simulink model "gm_inc_enc_v25_vnl"  (R2022a)
settings: Solver=FixedStepDiscrete  StartTime=0.0  StopTime=SimulationsDauer  RelTol=1e-3
undefined symbols (not defined in the file or in its folder): DiscIntNeverNeededParam, f_ISR, IncPerTurn, inital_zero_speed_timeout, n_max, OmegaPerOverSampl, Periode, Phase_Delay_A, Phase_Delay_B, PolePair, QuadratureFactor, reciprocal_iterations, T_fpga, T_mech
libraries: simulink x19, hdlsllib x11, hdlmdlgenlib x4, dspsrcs4 x3, dspswit3 x2, spsEdgeDetectorLib x2, simulink_extras x1
(part 2 of 4)

== system gm_inc_enc_v25_vnl/Compare/Assert_theta_el ==
  cosim : Inport
  dut : Inport  Port=2
  AssertEq : Assertion  StopWhenAssertionFail=off
  Compare To Zero : simulink/Logic and Bit Operations/Compare To Zero  relop===  OutDataTypeStr=boolean
  Relational Operator : RelationalOperator  Operator===  OutDataTypeStr=boolean  InputSameDT=off
  compare: theta_el : Scope  NumInputPorts=3
  wires:
  Compare To Zero/1 -> compare: theta_el/3  "err"
  Relational Operator/1 -> Compare To Zero/1, AssertEq/1
  cosim/1 -> compare: theta_el/1, Relational Operator/1  "cosim"
  dut/1 -> compare: theta_el/2, Relational Operator/2  "dut ref"

== system gm_inc_enc_v25_vnl/Compare/Assert_theta_el_AXI4 ==
  cosim : Inport
  dut : Inport  Port=2
  AssertEq : Assertion  StopWhenAssertionFail=off
  Compare To Zero : simulink/Logic and Bit Operations/Compare To Zero  relop===  OutDataTypeStr=boolean
  Relational Operator : RelationalOperator  Operator===  OutDataTypeStr=boolean  InputSameDT=off
  compare: theta_el_AXI4 : Scope  NumInputPorts=3
  wires:
  Compare To Zero/1 -> compare: theta_el_AXI4/3  "err"
  Relational Operator/1 -> Compare To Zero/1, AssertEq/1
  cosim/1 -> compare: theta_el_AXI4/1, Relational Operator/1  "cosim"
  dut/1 -> compare: theta_el_AXI4/2, Relational Operator/2  "dut ref"

== system gm_inc_enc_v25_vnl/Compare/Assert_timeout_active ==
  cosim : Inport
  dut : Inport  Port=2
  AssertEq : Assertion  StopWhenAssertionFail=off
  Compare To Zero : simulink/Logic and Bit Operations/Compare To Zero  relop===  OutDataTypeStr=boolean
  Relational Operator : RelationalOperator  Operator===  OutDataTypeStr=boolean  InputSameDT=off
  compare: timeout_active : Scope  NumInputPorts=3
  wires:
  Compare To Zero/1 -> compare: timeout_active/3  "err"
  Relational Operator/1 -> Compare To Zero/1, AssertEq/1
  cosim/1 -> compare: timeout_active/1, Relational Operator/1  "cosim"
  dut/1 -> compare: timeout_active/2, Relational Operator/2  "dut ref"

== system gm_inc_enc_v25_vnl/Compare/CleanupScopes ==

== system gm_inc_enc_v25_vnl/Compare/Enable ==

== system gm_inc_enc_v25_vnl/IncEnc_V25/Counter ==
  note: 1 for one cycle if edge recognized
  note: Reset
  Enable_ctr : Inport  OutDataTypeStr=boolean  PortDimensions=1  SampleTime=1e-08
  I_line : Inport  Port=2  OutDataTypeStr=boolean  PortDimensions=1  SampleTime=1e-08
  Detec_edge : Sum  Inputs=+-  AccumDataTypeStr=int8  OutDataTypeStr=int8  SampleTime=1e-08
  Reset_flag : Sum  Inputs=+-  AccumDataTypeStr=uint8  OutDataTypeStr=uint8  SampleTime=1e-08
  reset_old : Delay  DelayLength=double(1)  InitialCondition=0  SampleTime=1e-08
  reset_old1 : Delay  DelayLength=double(1)  InitialCondition=0  SampleTime=1e-08
  reset_old_switch : Switch  Criteria=u2 ~= 0  Threshold=double(0)  OutDataTypeStr=boolean  SampleTime=1e-08  SaturateOnIntegerOverflow=off  InputSameDT=off
  reset_old_switch1 : Switch  Criteria=u2 ~= 0  Threshold=double(0)  OutDataTypeStr=boolean  SampleTime=1e-08  SaturateOnIntegerOverflow=off  InputSameDT=off
  Edge : Outport  SampleTime=1e-08  VectorParamsAs1DForOutWhenUnconnected=off
  Reset : Outport  Port=2  SampleTime=1e-08  VectorParamsAs1DForOutWhenUnconnected=off
  wires:
  reset_old/1 -> Reset_flag/2, reset_old_switch/3
  reset_old_switch/1 -> reset_old/1
  reset_old1/1 -> Detec_edge/2, reset_old_switch1/3
  reset_old_switch1/1 -> reset_old1/1
  Reset_flag/1 -> reset_old_switch/2, Reset/1
  Detec_edge/1 -> reset_old_switch1/2, Edge/1
  I_line/1 -> reset_old_switch/1, Reset_flag/1
  Enable_ctr/1 -> reset_old_switch1/1, Detec_edge/1

== system gm_inc_enc_v25_vnl/IncEnc_V25/Counter_position ==
  note: Count
  note: Check if count is to big 0-Increments
  note: Check if count is to small
  Edge : Inport  OutDataTypeStr=int8  PortDimensions=1  SampleTime=1e-08
  Reset : Inport  Port=2  OutDataTypeStr=uint8  PortDimensions=1  SampleTime=1e-08
  IncsPerTurn : Inport  Port=3  OutDataTypeStr=uint16  PortDimensions=1  SampleTime=1e-08
  Dir : Inport  Port=4  OutDataTypeStr=fixdt(1, 4, 0)  PortDimensions=1  SampleTime=1e-08
  Add1 : Sum  AccumDataTypeStr=int16  OutDataTypeStr=int16  SampleTime=1e-08
  Constant1 : Constant  Value=0  OutDataTypeStr=int16  SampleTime=1e-08
  Constant2 : Constant  OutDataTypeStr=int16  SampleTime=1e-08
  Constant3 : Constant  Value=0  OutDataTypeStr=int16  SampleTime=1e-08
  Constant5 : Constant  Value=-1  OutDataTypeStr=int16  SampleTime=1e-08
  Relational Operator : RelationalOperator  Operator=>  OutDataTypeStr=boolean  SampleTime=1e-08  InputSameDT=off
  Relational Operator1 : RelationalOperator  Operator=<=  OutDataTypeStr=boolean  SampleTime=1e-08  InputSameDT=off
  Resett_switch1 : Switch  Criteria=u2 ~= 0  Threshold=double(0)  OutDataTypeStr=uint16  SampleTime=1e-08  SaturateOnIntegerOverflow=off  InputSameDT=off
  Resett_switch2 : Switch  Criteria=u2 ~= 0  Threshold=double(0)  OutDataTypeStr=int16  SampleTime=1e-08  SaturateOnIntegerOverflow=off  InputSameDT=off
  Resett_switch3 : Switch  Criteria=u2 ~= 0  Threshold=double(0)  OutDataTypeStr=int16  SampleTime=1e-08  SaturateOnIntegerOverflow=off  InputSameDT=off
  only_use_for_neg_speed : Switch  Threshold=double(1)  OutDataTypeStr=int16  SampleTime=1e-08  SaturateOnIntegerOverflow=off  InputSameDT=off
  reset_old{1..6} (6 alike) : Delay  DelayLength=double(1)  InitialCondition=0  SampleTime=1e-08
  speed_old_switch1 : Switch  Criteria=u2 ~= 0  Threshold=double(0)  OutDataTypeStr=int16  SampleTime=1e-08  SaturateOnIntegerOverflow=off  InputSameDT=off
  speed_old_switch2 : Switch  Threshold=double(1)  OutDataTypeStr=int16  SampleTime=1e-08  SaturateOnIntegerOverflow=off  InputSameDT=off
  count : Outport  SampleTime=1e-08  VectorParamsAs1DForOutWhenUnconnected=off
  wires:
  reset_old3/1 -> Resett_switch1/2
  Relational Operator/1 -> reset_old3/1
  Resett_switch3/1 -> Relational Operator1/1, Resett_switch1/3
  only_use_for_neg_speed/1 -> Resett_switch3/2
  reset_old2/1 -> only_use_for_neg_speed/3
  Relational Operator1/1 -> reset_old2/1
  reset_old1/1 -> Add1/2
  Add1/1 -> Resett_switch2/3
  Resett_switch2/1 -> Resett_switch3/3
  speed_old_switch2/1 -> reset_old4/1
  speed_old_switch1/1 -> Add1/1
  reset_old6/1 -> only_use_for_neg_speed/2, speed_old_switch2/2
  reset_old5/1 -> Resett_switch3/1, Relational Operator/2
  reset_old4/1 -> speed_old_switch1/1
  Resett_switch1/1 -> Relational Operator/1, reset_old1/1, count/1
  Constant5/1 -> speed_old_switch2/3
  Constant3/1 -> speed_old_switch1/3
  Constant2/1 -> speed_old_switch2/1
  Constant1/1 -> only_use_for_neg_speed/1, Resett_switch2/1, Resett_switch1/1, Relational Operator1/2
  Dir/1 -> reset_old6/1
  IncsPerTurn/1 -> reset_old5/1
  Reset/1 -> Resett_switch2/2
  Edge/1 -> speed_old_switch1/2

== system gm_inc_enc_v25_vnl/IncEnc_V25/Counter_theta_ele ==
  note: Count
  note: Check if count is to small
  Edge : Inport  OutDataTypeStr=int8  PortDimensions=1  SampleTime=1e-08
  Reset : Inport  Port=2  OutDataTypeStr=uint8  PortDimensions=1  SampleTime=1e-08
  IncsPerTurn : Inport  Port=3  OutDataTypeStr=uint16  PortDimensions=1  SampleTime=1e-08
  Dir : Inport  Port=4  OutDataTypeStr=fixdt(1, 4, 0)  PortDimensions=1  SampleTime=1e-08
  Add1 : Sum  AccumDataTypeStr=int16  OutDataTypeStr=int16  SampleTime=1e-08
  Constant1 : Constant  Value=0  OutDataTypeStr=int16  SampleTime=1e-08
  Constant2 : Constant  OutDataTypeStr=int16  SampleTime=1e-08
  Constant3 : Constant  Value=0  OutDataTypeStr=int16  SampleTime=1e-08
  Constant5 : Constant  Value=-1  OutDataTypeStr=int16  SampleTime=1e-08
  Relational Operator : RelationalOperator  Operator=>  OutDataTypeStr=boolean  SampleTime=1e-08  InputSameDT=off
  Relational Operator1 : RelationalOperator  Operator=<=  OutDataTypeStr=boolean  SampleTime=1e-08  InputSameDT=off
  Reset_switch3 : Switch  Criteria=u2 ~= 0  Threshold=double(0)  OutDataTypeStr=int16  SampleTime=1e-08  SaturateOnIntegerOverflow=off  InputSameDT=off
  Resett_switch1 : Switch  Criteria=u2 ~= 0  Threshold=double(0)  OutDataTypeStr=int16  SampleTime=1e-08  SaturateOnIntegerOverflow=off  InputSameDT=off
  Resett_switch2 : Switch  Criteria=u2 ~= 0  Threshold=double(0)  OutDataTypeStr=int16  SampleTime=1e-08  SaturateOnIntegerOverflow=off  InputSameDT=off
  only_use_for_neg_speed : Switch  Threshold=double(1)  OutDataTypeStr=int16  SampleTime=1e-08  SaturateOnIntegerOverflow=off  InputSameDT=off
  reset_old{1..6} (6 alike) : Delay  DelayLength=double(1)  InitialCondition=0  SampleTime=1e-08
  speed_old_switch1 : Switch  Criteria=u2 ~= 0  Threshold=double(0)  OutDataTypeStr=int16  SampleTime=1e-08  SaturateOnIntegerOverflow=off  InputSameDT=off
  speed_old_switch2 : Switch  Threshold=double(1)  OutDataTypeStr=int16  SampleTime=1e-08  SaturateOnIntegerOverflow=off  InputSameDT=off
  count : Outport  SampleTime=1e-08  VectorParamsAs1DForOutWhenUnconnected=off
  wires:
  reset_old3/1 -> Resett_switch1/2
  Relational Operator/1 -> reset_old3/1
  Reset_switch3/1 -> Relational Operator1/1, Resett_switch1/3
  only_use_for_neg_speed/1 -> Reset_switch3/2
  reset_old2/1 -> only_use_for_neg_speed/3
  Relational Operator1/1 -> reset_old2/1
  reset_old6/1 -> Add1/2
  Add1/1 -> Resett_switch2/3
  Resett_switch2/1 -> Reset_switch3/3
  speed_old_switch2/1 -> reset_old4/1
  speed_old_switch1/1 -> Add1/1
  reset_old5/1 -> only_use_for_neg_speed/2, speed_old_switch2/2
  reset_old4/1 -> speed_old_switch1/1
  reset_old1/1 -> Reset_switch3/1, Relational Operator/2
  Resett_switch1/1 -> Relational Operator/1, reset_old6/1, count/1
  Constant5/1 -> speed_old_switch2/3
  Constant3/1 -> speed_old_switch1/3
  Constant2/1 -> speed_old_switch2/1
  Constant1/1 -> only_use_for_neg_speed/1, Resett_switch2/1, Resett_switch1/1, Relational Operator1/2
  Dir/1 -> reset_old5/1
  IncsPerTurn/1 -> reset_old1/1
  Reset/1 -> Resett_switch2/2
  Edge/1 -> speed_old_switch1/2

== system gm_inc_enc_v25_vnl/IncEnc_V25/Direction ==
  A : Inport  OutDataTypeStr=boolean  PortDimensions=1  SampleTime=1e-08
  B : Inport  Port=2  OutDataTypeStr=boolean  PortDimensions=1  SampleTime=1e-08
  Add : Sum  Inputs=+-  AccumDataTypeStr=fixdt(1, 4, 0)  OutDataTypeStr=fixdt(1, 4, 0)  SampleTime=1e-08
  Add1 : Sum  Inputs=+-  AccumDataTypeStr=fixdt(1, 4, 0)  OutDataTypeStr=fixdt(1, 4, 0)  SampleTime=1e-08
  Add2 : Sum  AccumDataTypeStr=fixdt(1, 4, 0)  OutDataTypeStr=fixdt(1, 4, 0)  SampleTime=1e-08
  Change : Sum  AccumDataTypeStr=fixdt(1, 4, 0)  OutDataTypeStr=fixdt(1, 4, 0)  SampleTime=1e-08
  Change1 : Delay  DelayLength=double(1)  InitialCondition=0  SampleTime=1e-08
  Save_Direction : Switch  Criteria=u2 ~= 0  Threshold=double(0)  OutDataTypeStr=fixdt(1, 4, 0)  SampleTime=1e-08  SaturateOnIntegerOverflow=off  InputSameDT=off
  T_count_switch : Switch  Threshold=double(1)  OutDataTypeStr=fixdt(1, 4, 0)  SampleTime=1e-08  SaturateOnIntegerOverflow=off  InputSameDT=off
  TrnLeft : Sum  Inputs=+-  AccumDataTypeStr=fixdt(1, 4, 0)  OutDataTypeStr=fixdt(1, 4, 0)  SampleTime=1e-08
  TrnRight : Sum  Inputs=+-  AccumDataTypeStr=fixdt(1, 4, 0)  OutDataTypeStr=fixdt(1, 4, 0)  SampleTime=1e-08
  TurnLeft : Constant  Value=-1  OutDataTypeStr=fixdt(1, 4, 0)  SampleTime=1e-08
  TurnRight : Constant  OutDataTypeStr=fixdt(1, 4, 0)  SampleTime=1e-08
  count_old : Delay  DelayLength=double(1)  InitialCondition=0  SampleTime=1e-08
  count_old1 : Delay  DelayLength=double(1)  InitialCondition=0  SampleTime=1e-08
  count_old2 : Delay  DelayLength=double(1)  InitialCondition=0  SampleTime=1e-08
  count_old_switch : Switch  Criteria=u2 ~= 0  Threshold=double(0)  OutDataTypeStr=boolean  SampleTime=1e-08  SaturateOnIntegerOverflow=off  InputSameDT=off
  count_old_switch1 : Switch  Criteria=u2 ~= 0  Threshold=double(0)  OutDataTypeStr=boolean  SampleTime=1e-08  SaturateOnIntegerOverflow=off  InputSameDT=off
  new_value : Delay  DelayLength=double(1)  InitialCondition=0  SampleTime=1e-08
  nothing : Constant  Value=0  OutDataTypeStr=fixdt(1, 4, 0)  SampleTime=1e-08
  nothing1 : Constant  Value=0  OutDataTypeStr=fixdt(1, 4, 0)  SampleTime=1e-08
  speed_old_switch : Switch  Threshold=double(1)  OutDataTypeStr=fixdt(1, 4, 0)  SampleTime=1e-08  SaturateOnIntegerOverflow=off  InputSameDT=off
  Dir : Outport  SampleTime=1e-08  VectorParamsAs1DForOutWhenUnconnected=off
  wires:
  Save_Direction/1 -> count_old2/1
  count_old1/1 -> Add1/2, count_old_switch1/3
  count_old_switch1/1 -> count_old1/1
  count_old/1 -> Add/2, count_old_switch/3
  count_old_switch/1 -> count_old/1
  speed_old_switch/1 -> Add2/2, Change/2
  nothing1/1 -> T_count_switch/3
  nothing/1 -> speed_old_switch/3
  new_value/1 -> Save_Direction/1
  count_old2/1 -> Save_Direction/3, Dir/1
  TurnRight/1 -> T_count_switch/1
  TurnLeft/1 -> speed_old_switch/1
  TrnRight/1 -> T_count_switch/2
  TrnLeft/1 -> speed_old_switch/2
  T_count_switch/1 -> Add2/1, Change/1
  Change1/1 -> Save_Direction/2
  Change/1 -> Change1/1
  Add2/1 -> new_value/1
  Add1/1 -> count_old_switch1/2, TrnLeft/1
  Add/1 -> count_old_switch/2, TrnRight/1
  B/1 -> count_old_switch1/1, Add1/1, TrnRight/2
  A/1 -> count_old_switch/1, Add/1, TrnLeft/2

== system gm_inc_enc_v25_vnl/IncEnc_V25/count_lines ==
  note: Set new counter value
  note: Check if count is to big in order to safe for value overflow
  note: Count
  Edge : Inport  OutDataTypeStr=int8  PortDimensions=1  SampleTime=1e-08
  Reset : Inport  Port=2  OutDataTypeStr=boolean  PortDimensions=1  SampleTime=1e-08
  IncsPerTurn : Inport  Port=3  OutDataTypeStr=uint16  PortDimensions=1  SampleTime=1e-08
  Add1 : Sum  AccumDataTypeStr=int16  OutDataTypeStr=int16  SampleTime=1e-08
  Constant1 : Constant  Value=0  OutDataTypeStr=int16  SampleTime=1e-08
  Constant2 : Constant  OutDataTypeStr=int16  SampleTime=1e-08
  Constant3 : Constant  Value=0  OutDataTypeStr=int16  SampleTime=1e-08
  Constant4 : Constant  Value=10  OutDataTypeStr=int16  SampleTime=1e-08
  Relational Operator : RelationalOperator  Operator=>  OutDataTypeStr=boolean  SampleTime=1e-08  InputSameDT=off
  Reset_when_overflow : Sum  AccumDataTypeStr=fixdt(1, 18, 0)  OutDataTypeStr=int16  SampleTime=1e-08
  Resett_switch1 : Switch  Criteria=u2 ~= 0  Threshold=double(0)  OutDataTypeStr=int16  SampleTime=1e-08  SaturateOnIntegerOverflow=off  InputSameDT=off
  Resett_switch2 : Switch  Criteria=u2 ~= 0  Threshold=double(0)  OutDataTypeStr=int16  SampleTime=1e-08  SaturateOnIntegerOverflow=off  InputSameDT=off
  reset_old{1,3..5} (4 alike) : Delay  DelayLength=double(1)  InitialCondition=0  SampleTime=1e-08
  reset_old_switch1 : Switch  Criteria=u2 ~= 0  Threshold=double(0)  OutDataTypeStr=int16  SampleTime=1e-08  SaturateOnIntegerOverflow=off  InputSameDT=off
  speed_old_switch1 : Switch  Criteria=u2 ~= 0  Threshold=double(0)  OutDataTypeStr=int16  SampleTime=1e-08  SaturateOnIntegerOverflow=off  InputSameDT=off
  count : Outport  SampleTime=1e-08  VectorParamsAs1DForOutWhenUnconnected=off
  wires:
  reset_old1/1 -> reset_old_switch1/3
  Resett_switch1/1 -> reset_old3/1
  Relational Operator/1 -> Resett_switch1/2
  Add1/1 -> Resett_switch2/3
  Resett_switch2/1 -> Resett_switch1/3
  speed_old_switch1/1 -> Add1/1
  reset_old_switch1/1 -> reset_old1/1, count/1
  reset_old5/1 -> Relational Operator/2
  reset_old4/1 -> speed_old_switch1/1
  reset_old3/1 -> reset_old_switch1/1, Relational Operator/1, Add1/2
  Reset_when_overflow/1 -> reset_old5/1
  Constant4/1 -> Reset_when_overflow/1
  Constant3/1 -> speed_old_switch1/3
  Constant2/1 -> reset_old4/1
  Constant1/1 -> Resett_switch2/1, Resett_switch1/1
  IncsPerTurn/1 -> Reset_when_overflow/2
  Reset/1 -> reset_old_switch1/2, Resett_switch2/2
  Edge/1 -> speed_old_switch1/2

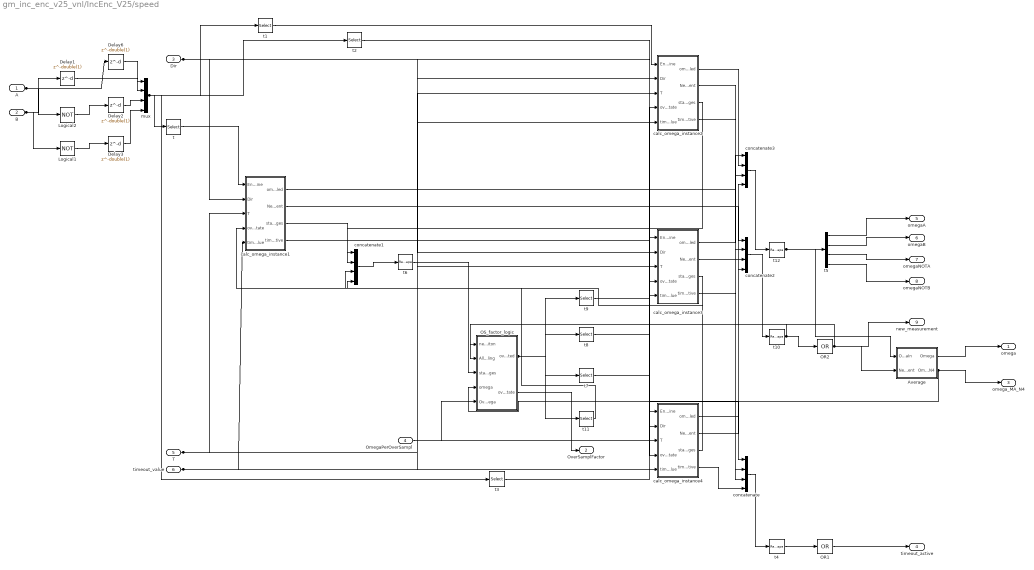
== system gm_inc_enc_v25_vnl/IncEnc_V25/speed ==
  A : Inport  OutDataTypeStr=boolean  PortDimensions=1  SampleTime=1e-08
  B : Inport  Port=2  OutDataTypeStr=boolean  PortDimensions=1  SampleTime=1e-08
  Dir : Inport  Port=3  OutDataTypeStr=fixdt(1, 4, 0)  PortDimensions=1  SampleTime=1e-08
  OmegaPerOverSampl : Inport  Port=4  OutDataTypeStr=fixdt(1, 24, 11)  PortDimensions=1  SampleTime=1e-08
  T : Inport  Port=5  OutDataTypeStr=fixdt(1, 38, 32)  PortDimensions=1  SampleTime=1e-08
  timeout_value : Inport  Port=6  OutDataTypeStr=uint32  PortDimensions=1  SampleTime=1e-08
  Average : Subsystem
  Delay{1..3,6} (4 alike) : Delay  DelayLength=double(1)  InitialCondition=0  SampleTime=1e-08
  Logical1 : Logic  Operator=NOT  Inputs=1  AllPortsSameDT=off  OutDataTypeStr=boolean  SampleTime=1e-08
  Logical2 : Logic  Operator=NOT  Inputs=1  AllPortsSameDT=off  OutDataTypeStr=boolean  SampleTime=1e-08
  OR1 : Logic  Operator=OR  Inputs=1  AllPortsSameDT=off  OutDataTypeStr=boolean  SampleTime=1e-08
  OR2 : Logic  Operator=OR  Inputs=1  AllPortsSameDT=off  OutDataTypeStr=boolean  SampleTime=1e-08
  OS_factor_logic : Subsystem
  calc_omega_instance1 : Subsystem
  calc_omega_instance2 : Subsystem
  calc_omega_instance3 : Subsystem
  calc_omega_instance4 : Subsystem
  concatenate{,1..3} (4 alike) : Concatenate  NumInputs=4
  mux : Mux
  t : Selector  SampleTime=1e-08  IndexOptions=Index vector (dialog)  Indices=double(1)  OutputSizes=1
  t1 : Selector  SampleTime=1e-08  IndexOptions=Index vector (dialog)  Indices=double(2)  OutputSizes=1
  t{4,6,10,12} (4 alike) : Reshape
  t11 : Selector  SampleTime=1e-08  IndexOptions=Index vector (dialog)  Indices=double(1)  OutputSizes=1
  t2 : Selector  SampleTime=1e-08  IndexOptions=Index vector (dialog)  Indices=double(3)  OutputSizes=1
  t3 : Selector  SampleTime=1e-08  IndexOptions=Index vector (dialog)  Indices=double(4)  OutputSizes=1
  t5 : Demux
  t7 : Selector  SampleTime=1e-08  IndexOptions=Index vector (dialog)  Indices=double(4)  OutputSizes=1
  t8 : Selector  SampleTime=1e-08  IndexOptions=Index vector (dialog)  Indices=double(3)  OutputSizes=1
  t9 : Selector  SampleTime=1e-08  IndexOptions=Index vector (dialog)  Indices=double(2)  OutputSizes=1
  omega : Outport  SampleTime=1e-08  VectorParamsAs1DForOutWhenUnconnected=off
  OverSamplFactor : Outport  Port=2  SampleTime=1e-08
  omega_MA_N4 : Outport  Port=3  SampleTime=1e-08  VectorParamsAs1DForOutWhenUnconnected=off
  timeout_active : Outport  Port=4  OutDataTypeStr=boolean  SampleTime=1e-08  VectorParamsAs1DForOutWhenUnconnected=off
  omegaA : Outport  Port=5  SampleTime=1e-08  VectorParamsAs1DForOutWhenUnconnected=off
  omegaB : Outport  Port=6  SampleTime=1e-08  VectorParamsAs1DForOutWhenUnconnected=off
  omegaNOTA : Outport  Port=7  SampleTime=1e-08  VectorParamsAs1DForOutWhenUnconnected=off
  omegaNOTB : Outport  Port=8  SampleTime=1e-08  VectorParamsAs1DForOutWhenUnconnected=off
  new_measurement : Outport  Port=9  OutDataTypeStr=boolean  SampleTime=1e-08  VectorParamsAs1DForOutWhenUnconnected=off
  wires:
  concatenate3/1 -> t12/1
  calc_omega_instance1/3(state_count_edges) -> concatenate1/1
  calc_omega_instance1/2(NewMeasurement) -> concatenate2/1
  calc_omega_instance1/1(omega_oversampled) -> concatenate3/1
  t11/1 -> calc_omega_instance1/4(oversampling_state)
  OS_factor_logic/1(oversampling_adjusted) -> t11/1, t9/1, t8/1, t7/1
  t10/1 -> OS_factor_logic/1(new_transisiton), OR2/1
  concatenate2/1 -> t10/1
  calc_omega_instance2/3(state_count_edges) -> concatenate1/2
  calc_omega_instance2/2(NewMeasurement) -> concatenate2/2
  calc_omega_instance2/1(omega_oversampled) -> concatenate3/2
  t9/1 -> calc_omega_instance2/4(oversampling_state)
  calc_omega_instance3/3(state_count_edges) -> concatenate1/3
  calc_omega_instance3/2(NewMeasurement) -> concatenate2/3
  calc_omega_instance3/1(omega_oversampled) -> concatenate3/3
  t8/1 -> calc_omega_instance3/4(oversampling_state)
  calc_omega_instance4/3(state_count_edges) -> concatenate1/4
  calc_omega_instance4/2(NewMeasurement) -> concatenate2/4
  calc_omega_instance4/1(omega_oversampled) -> concatenate3/4
  t7/1 -> calc_omega_instance4/4(oversampling_state)
  t6/1 -> OS_factor_logic/3(state_edges)
  concatenate1/1 -> t6/1
  t5/4 -> omegaNOTB/1
  t5/3 -> omegaNOTA/1
  t5/2 -> omegaB/1
  t5/1 -> omegaA/1
  calc_omega_instance4/4(timeout_active) -> concatenate/4
  calc_omega_instance3/4(timeout_active) -> concatenate/3
  calc_omega_instance2/4(timeout_active) -> concatenate/2
  calc_omega_instance1/4(timeout_active) -> concatenate/1
  concatenate/1 -> t4/1
  t3/1 -> calc_omega_instance4/1(Encoder Line)
  t2/1 -> calc_omega_instance3/1(Encoder Line)
  t1/1 -> calc_omega_instance2/1(Encoder Line)
  t/1 -> calc_omega_instance1/1(Encoder Line)
  t4/1 -> OR1/1
  t12/1 -> Average/1("OmegaIn "), t5/1
  OS_factor_logic/2(oversampling_state) -> OverSamplFactor/1
  OR2/1 -> OS_factor_logic/2(Allow_ToCheckOversampling), Average/2(NewMeasurement), new_measurement/1
  OR1/1 -> timeout_active/1
  mux/1 -> t/1, t1/1, t2/1, t3/1
  Logical2/1 -> Delay2/1
  Logical1/1 -> Delay3/1
  Delay6/1 -> mux/1
  Delay3/1 -> mux/4
  Delay2/1 -> mux/3
  Delay1/1 -> mux/2
  Average/2(OmegaOut_MA_N4) -> OS_factor_logic/4(omega), omega_MA_N4/1
  Average/1(Omega) -> omega/1
  timeout_value/1 -> calc_omega_instance4/5(timeout_value), calc_omega_instance3/5(timeout_value), calc_omega_instance2/5(timeout_value), calc_omega_instance1/5(timeout_value)
  T/1 -> calc_omega_instance4/3(T), calc_omega_instance3/3(T), calc_omega_instance2/3(T), calc_omega_instance1/3(T)
  OmegaPerOverSampl/1 -> OS_factor_logic/5(OverSamplOmega)
  Dir/1 -> calc_omega_instance4/2(Dir), calc_omega_instance3/2(Dir), calc_omega_instance2/2(Dir), calc_omega_instance1/2(Dir)
  B/1 -> Delay1/1, Logical1/1
  A/1 -> Delay6/1, Logical2/1

== system gm_inc_enc_v25_vnl/IncEnc_V25_vnl/Counter ==
  note: Reset
  note: 1 for one cycle if edge recognized
  Enable_ctr : Inport
  I_line : Inport  Port=2
  Detec_edge : Sum  Inputs=+-  AccumDataTypeStr=int8  OutDataTypeStr=int8
  Reset_flag : Sum  Inputs=+-  AccumDataTypeStr=uint8  OutDataTypeStr=uint8
  reset_old : Delay  DelayLength=1
  reset_old1 : Delay  DelayLength=1
  reset_old_switch : Switch  Criteria=u2 ~= 0  SaturateOnIntegerOverflow=off  InputSameDT=off
  reset_old_switch1 : Switch  Criteria=u2 ~= 0  SaturateOnIntegerOverflow=off  InputSameDT=off
  Edge : Outport  VectorParamsAs1DForOutWhenUnconnected=off
  Reset : Outport  Port=2  VectorParamsAs1DForOutWhenUnconnected=off
  wires:
  Detec_edge/1 -> Edge/1, reset_old_switch1/2  "1 for one cycle if edge recognized"
  reset_old1/1 -> Detec_edge/2, reset_old_switch1/3
  reset_old_switch1/1 -> reset_old1/1
  Enable_ctr/1 -> reset_old_switch1/1, Detec_edge/1
  Reset_flag/1 -> reset_old_switch/2, Reset/1
  reset_old/1 -> Reset_flag/2, reset_old_switch/3
  reset_old_switch/1 -> reset_old/1
  I_line/1 -> reset_old_switch/1, Reset_flag/1

== system gm_inc_enc_v25_vnl/IncEnc_V25_vnl/Counter_position ==
  note: Check if count is to small
  note: Check if count is to big 0-Increments
  note: Count
  Edge : Inport
  Reset : Inport  Port=2
  IncsPerTurn : Inport  Port=3
  Dir : Inport  Port=4
  Add1 : Sum  AccumDataTypeStr=int16  OutDataTypeStr=int16
  Constant1 : Constant  Value=0  OutDataTypeStr=int16  SampleTime=-1
  Constant2 : Constant  OutDataTypeStr=int16  SampleTime=-1
  Constant3 : Constant  Value=0  OutDataTypeStr=int16  SampleTime=-1
  Constant5 : Constant  Value=-1  OutDataTypeStr=int16  SampleTime=-1
  Relational Operator : RelationalOperator  Operator=>  OutDataTypeStr=boolean  InputSameDT=off
  Relational Operator1 : RelationalOperator  Operator=<=  OutDataTypeStr=boolean  InputSameDT=off
  Resett_switch1 : Switch  Criteria=u2 ~= 0  OutDataTypeStr=uint16  SaturateOnIntegerOverflow=off  InputSameDT=off
  Resett_switch2 : Switch  Criteria=u2 ~= 0  OutDataTypeStr=int16  SaturateOnIntegerOverflow=off  InputSameDT=off
  Resett_switch3 : Switch  Criteria=u2 ~= 0  OutDataTypeStr=int16  SaturateOnIntegerOverflow=off  InputSameDT=off
  only_use_for_neg_speed : Switch  Threshold=1  SaturateOnIntegerOverflow=off  InputSameDT=off
  reset_old{1..6} (6 alike) : Delay  DelayLength=1
  speed_old_switch1 : Switch  Criteria=u2 ~= 0  SaturateOnIntegerOverflow=off  InputSameDT=off
  speed_old_switch2 : Switch  Threshold=1  SaturateOnIntegerOverflow=off  InputSameDT=off
  count : Outport  VectorParamsAs1DForOutWhenUnconnected=off
  wires:
  reset_old1/1 -> Add1/2
  reset_old5/1 -> Resett_switch3/1, Relational Operator/2
  reset_old2/1 -> only_use_for_neg_speed/3
  reset_old3/1 -> Resett_switch1/2
  Resett_switch1/1 -> count/1, reset_old1/1, Relational Operator/1
  reset_old6/1 -> speed_old_switch2/2, only_use_for_neg_speed/2
  IncsPerTurn/1 -> reset_old5/1
  reset_old4/1 -> speed_old_switch1/1
  only_use_for_neg_speed/1 -> Resett_switch3/2
  Relational Operator1/1 -> reset_old2/1
  Resett_switch3/1 -> Resett_switch1/3, Relational Operator1/1
  Resett_switch2/1 -> Resett_switch3/3
  Constant1/1 -> Resett_switch2/1, Relational Operator1/2, only_use_for_neg_speed/1, Resett_switch1/1
  Relational Operator/1 -> reset_old3/1
  speed_old_switch2/1 -> reset_old4/1
  Constant5/1 -> speed_old_switch2/3
  Dir/1 -> reset_old6/1
  Constant2/1 -> speed_old_switch2/1
  Constant3/1 -> speed_old_switch1/3
  speed_old_switch1/1 -> Add1/1
  Add1/1 -> Resett_switch2/3
  Edge/1 -> speed_old_switch1/2  "1 for one cycle if edge recognized"
  Reset/1 -> Resett_switch2/2

== system gm_inc_enc_v25_vnl/IncEnc_V25_vnl/Counter_theta_ele ==
  note: Check if count is to small
  note: Check if count is to big
      | -Count from 0-Increments
      | - e.g. for 5000 increments, 4 pole pairs and A/B-Line (quadrature),
      | we count from 0-(5000*4/4) = 0-5000
      | - In that case, we must reset to 0, as soon as we have a value,
      | which is 1 bigger than increments (e.g. 5001 = 0).
  note: Count
  note: This Reset (I-Line) synchronize only
      | theta with position.
      | Since I-Line comes only once per
      | mechanical turn. Normaly the "IncsPerTurn"
      | do the Reset.
  Edge : Inport
  Reset : Inport  Port=2
  IncsPerTurn : Inport  Port=3
  Dir : Inport  Port=4
  Add1 : Sum  AccumDataTypeStr=int16  OutDataTypeStr=int16
  Constant1 : Constant  Value=0  OutDataTypeStr=int16  SampleTime=-1
  Constant2 : Constant  OutDataTypeStr=int16  SampleTime=-1
  Constant3 : Constant  Value=0  OutDataTypeStr=int16  SampleTime=-1
  Constant5 : Constant  Value=-1  OutDataTypeStr=int16  SampleTime=-1
  Relational Operator : RelationalOperator  Operator=>  OutDataTypeStr=boolean  InputSameDT=off
  Relational Operator1 : RelationalOperator  Operator=<=  OutDataTypeStr=boolean  InputSameDT=off
  Reset_switch3 : Switch  Criteria=u2 ~= 0  OutDataTypeStr=int16  SaturateOnIntegerOverflow=off  InputSameDT=off
  Resett_switch1 : Switch  Criteria=u2 ~= 0  OutDataTypeStr=int16  SaturateOnIntegerOverflow=off  InputSameDT=off
  Resett_switch2 : Switch  Criteria=u2 ~= 0  OutDataTypeStr=int16  SaturateOnIntegerOverflow=off  InputSameDT=off
  only_use_for_neg_speed : Switch  Threshold=1  SaturateOnIntegerOverflow=off  InputSameDT=off
  reset_old{1..6} (6 alike) : Delay  DelayLength=1
  speed_old_switch1 : Switch  Criteria=u2 ~= 0  SaturateOnIntegerOverflow=off  InputSameDT=off
  speed_old_switch2 : Switch  Threshold=1  SaturateOnIntegerOverflow=off  InputSameDT=off
  count : Outport  VectorParamsAs1DForOutWhenUnconnected=off
  wires:
  reset_old6/1 -> Add1/2
  reset_old1/1 -> Reset_switch3/1, Relational Operator/2
  reset_old2/1 -> only_use_for_neg_speed/3
  reset_old3/1 -> Resett_switch1/2
  reset_old5/1 -> only_use_for_neg_speed/2, speed_old_switch2/2
  reset_old4/1 -> speed_old_switch1/1
  only_use_for_neg_speed/1 -> Reset_switch3/2
  Relational Operator1/1 -> reset_old2/1
  Reset_switch3/1 -> Resett_switch1/3, Relational Operator1/1
  Resett_switch2/1 -> Reset_switch3/3
  Constant1/1 -> Resett_switch1/1, Relational Operator1/2, only_use_for_neg_speed/1, Resett_switch2/1
  Relational Operator/1 -> reset_old3/1
  Resett_switch1/1 -> Relational Operator/1, count/1, reset_old6/1
  speed_old_switch2/1 -> reset_old4/1
  Constant5/1 -> speed_old_switch2/3
  Dir/1 -> reset_old5/1
  IncsPerTurn/1 -> reset_old1/1
  Constant2/1 -> speed_old_switch2/1
  Constant3/1 -> speed_old_switch1/3
  speed_old_switch1/1 -> Add1/1
  Add1/1 -> Resett_switch2/3
  Edge/1 -> speed_old_switch1/2  "1 for one cycle if edge recognized"
  Reset/1 -> Resett_switch2/2

== system gm_inc_enc_v25_vnl/IncEnc_V25_vnl/Direction ==
  A : Inport
  B : Inport  Port=2
  Add : Sum  Inputs=+-  AccumDataTypeStr=fixdt(1,4,0)  OutDataTypeStr=fixdt(1,4,0)
  Add1 : Sum  Inputs=+-  AccumDataTypeStr=fixdt(1,4,0)  OutDataTypeStr=fixdt(1,4,0)
  Add2 : Sum  AccumDataTypeStr=fixdt(1,4,0)  OutDataTypeStr=fixdt(1,4,0)
  Change : Sum  AccumDataTypeStr=fixdt(1,4,0)  OutDataTypeStr=fixdt(1,4,0)
  Change1 : Delay  DelayLength=1
  Save_Direction : Switch  Criteria=u2 ~= 0  Threshold=0.1  OutDataTypeStr=fixdt(1,4,0)  SaturateOnIntegerOverflow=off  InputSameDT=off
  T_count_switch : Switch  Threshold=1  OutDataTypeStr=Inherit: Inherit via back propagation  SaturateOnIntegerOverflow=off  InputSameDT=off
  TrnLeft : Sum  Inputs=+-  AccumDataTypeStr=fixdt(1,4,0)  OutDataTypeStr=fixdt(1,4,0)
  TrnRight : Sum  Inputs=+-  AccumDataTypeStr=fixdt(1,4,0)  OutDataTypeStr=fixdt(1,4,0)
  TurnLeft : Constant  Value=-1  OutDataTypeStr=fixdt(1,4,0)  SampleTime=-1
  TurnRight : Constant  OutDataTypeStr=fixdt(1,4,0)  SampleTime=-1
  count_old : Delay  DelayLength=1
  count_old1 : Delay  DelayLength=1
  count_old2 : Delay  DelayLength=1
  count_old_switch : Switch  Criteria=u2 ~= 0  OutDataTypeStr=Inherit: Inherit via back propagation  SaturateOnIntegerOverflow=off  InputSameDT=off
  count_old_switch1 : Switch  Criteria=u2 ~= 0  OutDataTypeStr=Inherit: Inherit via back propagation  SaturateOnIntegerOverflow=off  InputSameDT=off
  new_value : Delay  DelayLength=1
  nothing : Constant  Value=0  OutDataTypeStr=fixdt(1,4,0)  SampleTime=-1
  nothing1 : Constant  Value=0  OutDataTypeStr=fixdt(1,4,0)  SampleTime=-1
  speed_old_switch : Switch  Threshold=1  OutDataTypeStr=Inherit: Inherit via back propagation  SaturateOnIntegerOverflow=off  InputSameDT=off
  Dir : Outport  VectorParamsAs1DForOutWhenUnconnected=off
  wires:
  count_old2/1 -> Dir/1, Save_Direction/3  "Dir"
  Change1/1 -> Save_Direction/2  "Change"
  Change/1 -> Change1/1
  Add2/1 -> new_value/1
  speed_old_switch/1 -> Add2/2, Change/2
  nothing1/1 -> T_count_switch/3
  nothing/1 -> speed_old_switch/3
  TurnLeft/1 -> speed_old_switch/1
  TrnLeft/1 -> speed_old_switch/2  "TrnLeft"
  new_value/1 -> Save_Direction/1
  TrnRight/1 -> T_count_switch/2  "Trn_Right"
  Add1/1 -> count_old_switch1/2, TrnLeft/1  "Edge_B"
  count_old1/1 -> Add1/2, count_old_switch1/3
  count_old_switch1/1 -> count_old1/1
  B/1 -> count_old_switch1/1, Add1/1, TrnRight/2
  Save_Direction/1 -> count_old2/1
  T_count_switch/1 -> Add2/1, Change/1
  Add/1 -> count_old_switch/2, TrnRight/1  "Edge_A"
  TurnRight/1 -> T_count_switch/1
  count_old/1 -> Add/2, count_old_switch/3
  count_old_switch/1 -> count_old/1
  A/1 -> count_old_switch/1, Add/1, TrnLeft/2

== system gm_inc_enc_v25_vnl/IncEnc_V25_vnl/count_lines ==
  note: omega by counting lines, can be used for high-speed, but is not recommended for small drives!
      | However, for using this approach, we need a quite long time window in order to get an accurate speed.
      | For small drives a long time window is not acceptable, since the mechanical time constant is small.
      | e.g. using just 100us (since the speed control has this period at 10kHz) we can calculate as following:
      | speed = 5034rpm, Increments = 5000, QuadratureFactor = 4, f_cc = 10000 kHz
      | In the test, 169 lines are counted in 100us in the described example.
      | -> 169*(10000/(4*5000))*60 = 5070rpm (so this is not accurate!)
      | However, a longer time window is not acceptabel for speed control with10kHz. More increments is not common, since 5000 are already a lot!
  note: Count
  note: Check if count is to big in order to safe for value overflow
  note: Set new counter value
  Edge : Inport
  Reset : Inport  Port=2
  IncsPerTurn : Inport  Port=3
  Add1 : Sum  AccumDataTypeStr=int16  OutDataTypeStr=int16
  Constant1 : Constant  Value=0  OutDataTypeStr=int16  SampleTime=-1
  Constant2 : Constant  OutDataTypeStr=int16  SampleTime=-1
  Constant3 : Constant  Value=0  OutDataTypeStr=int16  SampleTime=-1
  Constant4 : Constant  Value=10  OutDataTypeStr=int16  SampleTime=-1
  Relational Operator : RelationalOperator  Operator=>  OutDataTypeStr=boolean  InputSameDT=off
  Reset_when_overflow : Sum  OutDataTypeStr=int16
  Resett_switch1 : Switch  Criteria=u2 ~= 0  OutDataTypeStr=int16  SaturateOnIntegerOverflow=off  InputSameDT=off
  Resett_switch2 : Switch  Criteria=u2 ~= 0  OutDataTypeStr=int16  SaturateOnIntegerOverflow=off  InputSameDT=off
  reset_old{1,3..5} (4 alike) : Delay  DelayLength=1
  reset_old_switch1 : Switch  Criteria=u2 ~= 0  SaturateOnIntegerOverflow=off  InputSameDT=off
  speed_old_switch1 : Switch  Criteria=u2 ~= 0  SaturateOnIntegerOverflow=off  InputSameDT=off
  count : Outport  VectorParamsAs1DForOutWhenUnconnected=off
  wires:
  reset_old_switch1/1 -> count/1, reset_old1/1
  Reset/1 -> Resett_switch2/2, reset_old_switch1/2  "Use new value"
  reset_old1/1 -> reset_old_switch1/3
  reset_old3/1 -> Relational Operator/1, Add1/2, reset_old_switch1/1
  Resett_switch1/1 -> reset_old3/1
  Constant4/1 -> Reset_when_overflow/1
  Constant2/1 -> reset_old4/1
  Add1/1 -> Resett_switch2/3
  IncsPerTurn/1 -> Reset_when_overflow/2
  Constant3/1 -> speed_old_switch1/3
  Constant1/1 -> Resett_switch1/1, Resett_switch2/1
  Edge/1 -> speed_old_switch1/2  "1 for one cycle if edge recognized"
  reset_old4/1 -> speed_old_switch1/1
  Resett_switch2/1 -> Resett_switch1/3
  reset_old5/1 -> Relational Operator/2
  speed_old_switch1/1 -> Add1/1
  Relational Operator/1 -> Resett_switch1/2
  Reset_when_overflow/1 -> reset_old5/1

== system gm_inc_enc_v25_vnl/IncEnc_V25_vnl/speed ==
  A : Inport
  B : Inport  Port=2
  Dir : Inport  Port=3
  OmegaPerOverSampl : Inport  Port=4
  T : Inport  Port=5
  timeout_value : Inport  Port=6  OutDataTypeStr=uint32
  Average : Subsystem
  Delay{1..3,6} (4 alike) : Delay  DelayLength=1  InitialCondition=0
  Demux : Demux
  Logical1 : Logic  Operator=NOT  AllPortsSameDT=off  OutDataTypeStr=boolean
  Logical2 : Logic  Operator=NOT  AllPortsSameDT=off  OutDataTypeStr=boolean
  Mux : Mux
  OR1 : Logic  Operator=OR  Inputs=1  AllPortsSameDT=off  OutDataTypeStr=boolean
  OR2 : Logic  Operator=OR  Inputs=1  AllPortsSameDT=off  OutDataTypeStr=boolean
  OS_factor_logic : Subsystem
      settings: PortSchema="{\"entries\":[{\"content\":{\"sides\":[{\"content\":{\"connectorIds\":[\"In1\",\"In2\",\"In3\",\"In4\",\"Out2\"]},\"type\":\"ConnectorPlacement.EquallySpacedRectSide\",\"uuid\":\"00190a63-1990-4dc8-8561-af6346041cd2\"},{\"content\":{\"connectorIds\":[\"Out1\",\"In5\"],\"side\":\"RIGHT\"},\"type\":\"ConnectorPlacement.EquallySpacedRectSide\",\"uuid\":\"ed8fa1bb-ba76-4f60-9676-d72d7f094a86\"},{\"content\":{\"connectorIds\":[],\"side\":\"TOP\"},\"type\":\"ConnectorPlacement.EquallySpacedRectSide\",\"uuid\":\"16aa4cab-6298-4523-a92b-d078d21511a0\"}]},\"type\":\"ConnectorPlacement.EquallySpacedConnector\",\"uuid\":\"bb0c721d-662f-49b4-b1e3-cc7ff0334cdb\"}],\"packageUris\":[\"http://schema.mathworks.com/mf0/Connector/R2020b\"],\"version\":\"1.0\"}"
  calc_omega : Subsystem  TreatAsAtomicUnit=on
  omega : Outport  VectorParamsAs1DForOutWhenUnconnected=off
  OverSamplFactor : Outport  Port=2
  omega_MA_N4 : Outport  Port=3  VectorParamsAs1DForOutWhenUnconnected=off
  timeout_active : Outport  Port=4  OutDataTypeStr=boolean  VectorParamsAs1DForOutWhenUnconnected=off
  omegaA : Outport  Port=5  VectorParamsAs1DForOutWhenUnconnected=off
  omegaB : Outport  Port=6  VectorParamsAs1DForOutWhenUnconnected=off
  omegaNOTA : Outport  Port=7  VectorParamsAs1DForOutWhenUnconnected=off
  omegaNOTB : Outport  Port=8  VectorParamsAs1DForOutWhenUnconnected=off
  new_measurement : Outport  Port=9  OutDataTypeStr=boolean  VectorParamsAs1DForOutWhenUnconnected=off
  wires:
  Average/1(Omega) -> omega/1
  Delay3/1 -> Mux/4
  Delay2/1 -> Mux/3
  Delay1/1 -> Mux/2
  Delay6/1 -> Mux/1
  OS_factor_logic/1(oversampling_adjusted) -> calc_omega/4(oversampling_state)
  Logical1/1 -> Delay3/1  "NOT_B"
  Logical2/1 -> Delay2/1  "NOT_A"
  calc_omega/4(timeout_active) -> OR1/1
  calc_omega/3(state_count_edges) -> OS_factor_logic/3(state_edges)
  calc_omega/2(NewMeasurement) -> OS_factor_logic/1(new_transisiton), OR2/1  "newMeas"
  calc_omega/1(omega_oversampled) -> Average/1("OmegaIn "), Demux/1  "omega"
  Demux/3 -> omegaNOTA/1
  Demux/4 -> omegaNOTB/1
  Demux/1 -> omegaA/1
  Demux/2 -> omegaB/1
  timeout_value/1 -> calc_omega/5(timeout_value)
  T/1 -> calc_omega/3(T)
  Mux/1 -> calc_omega/1(Encoder Line)
  A/1 -> Delay6/1, Logical2/1  "A"
  Average/2(OmegaOut_MA_N4) -> OS_factor_logic/4(omega), omega_MA_N4/1  "final omega oversampled"
  OR1/1 -> timeout_active/1  "timeout_active_all_ORed"
  OS_factor_logic/2(oversampling_state) -> OverSamplFactor/1  "OS_B"
  OR2/1 -> new_measurement/1, Average/2(NewMeasurement), OS_factor_logic/2(Allow_ToCheckOversampling)  "newMeas_allORed"
  OmegaPerOverSampl/1 -> OS_factor_logic/5(OverSamplOmega)
  B/1 -> Logical1/1, Delay1/1  "B"
  Dir/1 -> calc_omega/2(Dir)

== system gm_inc_enc_v25_vnl/IncrementalEncoder_Floating/CutTheta_0_2PI ==
  In1 : Inport
  Add7 : Sum  Inputs=+-  OutDataTypeStr=double
  Gain : Gain  Gain=1/(2*pi)
  Gain11 : Gain  Gain=2*pi
  Rounding Function : Rounding
  Out1 : Outport  VectorParamsAs1DForOutWhenUnconnected=off
  wires:
  Gain/1 -> Rounding Function/1
  Rounding Function/1 -> Gain11/1
  Gain11/1 -> Add7/2
  In1/1 -> Gain/1, Add7/1
  Add7/1 -> Out1/1

== system gm_inc_enc_v25_vnl/IncrementalEncoder_Floating/n_aus_theta_v4 ==
  theta : Inport
  Abs : Abs  SaturateOnIntegerOverflow=off
  Add : Sum  Inputs=-+
  Add1 : Sum  Inputs=+-
  Gain : Gain  Gain=2*pi
  Gain1 : Gain  Gain=1/T_mech
  Gain2 : Gain  Gain=60/(2*pi)
  Geschwindigkeitsfilter1 : Subsystem
  Rate Limiter2 1/T : RateLimiter  RisingSlewLimit=1/T_mech*10  FallingSlewLimit=-1/T_mech*10  SampleTimeMode=inherited
  Saturation : Saturate  UpperLimit=n_max  LowerLimit=-n_max
  Scope1 : Scope  NumInputPorts=5
  Scope2 : Scope  NumInputPorts=5
  Sign : Signum
  Switch : Switch  Threshold=3  SaturateOnIntegerOverflow=off  InputSameDT=off
  Unit Delay : UnitDelay  SampleTime=-1  HasFrameUpgradeWarning=on
  n : Outport  VectorParamsAs1DForOutWhenUnconnected=off
  wires:
  Switch/1 -> Scope1/3, Gain1/1
  Add/1 -> Scope2/1, Switch/1
  Gain/1 -> Add/1
  Sign/1 -> Gain/1
  Add1/1 -> Scope2/3, Add/2, Abs/1, Scope2/2, Switch/3, Sign/1
  Abs/1 -> Scope1/4, Switch/2
  Gain1/1 -> Scope1/2, Gain2/1
  theta/1 -> Scope2/5, Add1/1, Unit Delay/1
  Unit Delay/1 -> Scope2/4, Add1/2
  Gain2/1 -> Saturation/1
  Geschwindigkeitsfilter1/1(Out1) -> Scope1/5, Rate Limiter2 1/T/1
  Rate Limiter2 1/T/1 -> n/1
  Saturation/1 -> Scope1/1, Geschwindigkeitsfilter1/1(In1)

== system gm_inc_enc_v25_vnl/IncEnc_V25/speed/Average ==
  note: average 4 parallel measurements
  note: moving average of 4 last measurements, which in total results in a moving average of the last 8 samples
  "OmegaIn " : Inport  OutDataTypeStr=fixdt(1, 24, 11)  PortDimensions=[4]  SampleTime=1e-08
  NewMeasurement : Inport  Port=2  OutDataTypeStr=boolean  PortDimensions=1  SampleTime=1e-08
  DelayToCompensate_sum : Delay  DelayLength=double(1)  InitialCondition=0  SampleTime=1e-08
  Gain : Gain  Gain="fi(0,1,26,26,\"hex\",\"1000000\")"  ParamDataTypeStr=fixdt(1, 26, 26)  OutDataTypeStr=fixdt(1, 24, 11)  SampleTime=1e-08
  Gain1 : Gain  Gain="fi(0,1,26,26,\"hex\",\"1000000\")"  ParamDataTypeStr=fixdt(1, 26, 26)  OutDataTypeStr=fixdt(1, 24, 11)  SampleTime=1e-08
  Sum of Elements{1..2,4..5} (4 alike) : Sum  AccumDataTypeStr=fixdt(1, 25, 11)  OutDataTypeStr=fixdt(1, 25, 11)  SampleTime=1e-08
  Sum of Elements3 : Sum  AccumDataTypeStr=fixdt(1, 26, 11)  OutDataTypeStr=fixdt(1, 26, 11)  SampleTime=1e-08
  Sum of Elements6 : Sum  AccumDataTypeStr=fixdt(1, 26, 11)  OutDataTypeStr=fixdt(1, 26, 11)  SampleTime=1e-08
  Unit Delay Enabled Synchronous : hdlsllib/Discrete/Unit Delay Enabled Synchronous  InitialCondition=double(0)  SampleTime=-1
      settings: SourceProductBaseCode=SL
  Unit Delay Enabled Synchronous1 : hdlsllib/Discrete/Unit Delay Enabled Synchronous  InitialCondition=double(0)  SampleTime=-1
      settings: SourceProductBaseCode=SL
  Unit Delay Enabled Synchronous2 : hdlsllib/Discrete/Unit Delay Enabled Synchronous  InitialCondition=double(0)  SampleTime=-1
      settings: SourceProductBaseCode=SL
  delay : Delay  DelayLength=double(1)  InitialCondition=0  SampleTime=1e-08
  delay1 : Delay  DelayLength=double(1)  InitialCondition=0  SampleTime=1e-08
  t : Demux
  x(k)_0_wire : hdlmdlgenlib/Buffer
      settings: SourceProductBaseCode=SL
  x(k)_1_wire : hdlmdlgenlib/Buffer
      settings: SourceProductBaseCode=SL
  x(k)_2_wire : hdlmdlgenlib/Buffer
      settings: SourceProductBaseCode=SL
  x(k)_3_wire : hdlmdlgenlib/Buffer
      settings: SourceProductBaseCode=SL
  Omega : Outport  SampleTime=1e-08  VectorParamsAs1DForOutWhenUnconnected=off
  OmegaOut_MA_N4 : Outport  Port=2  SampleTime=1e-08  VectorParamsAs1DForOutWhenUnconnected=off
  wires:
  NewMeasurement/1 -> delay/1
  "OmegaIn "/1 -> t/1
  t/4 -> x(k)_3_wire/1
  t/3 -> x(k)_2_wire/1
  t/2 -> x(k)_1_wire/1
  t/1 -> x(k)_0_wire/1
  delay1/1 -> Sum of Elements1/1
  delay/1 -> Unit Delay Enabled Synchronous/2, Unit Delay Enabled Synchronous1/2, Unit Delay Enabled Synchronous2/2
  Unit Delay Enabled Synchronous2/1 -> Sum of Elements2/2
  Unit Delay Enabled Synchronous1/1 -> Unit Delay Enabled Synchronous2/1, Sum of Elements2/1
  Unit Delay Enabled Synchronous/1 -> Unit Delay Enabled Synchronous1/1, Sum of Elements1/2
  Sum of Elements6/1 -> Gain1/1
  Sum of Elements5/1 -> Sum of Elements6/2
  Sum of Elements4/1 -> Sum of Elements6/1
  Sum of Elements3/1 -> Gain/1
  Sum of Elements2/1 -> Sum of Elements3/2
  Sum of Elements1/1 -> Sum of Elements3/1
  Gain1/1 -> DelayToCompensate_sum/1
  Gain/1 -> OmegaOut_MA_N4/1
  x(k)_3_wire/1 -> Sum of Elements5/2
  x(k)_2_wire/1 -> Sum of Elements5/1
  x(k)_1_wire/1 -> Sum of Elements4/2
  x(k)_0_wire/1 -> Sum of Elements4/1
  DelayToCompensate_sum/1 -> Omega/1, Unit Delay Enabled Synchronous/1, delay1/1

== system gm_inc_enc_v25_vnl/IncEnc_V25/speed/OS_factor_logic ==
  new_transisiton : Inport  OutDataTypeStr=boolean  PortDimensions=[4]  SampleTime=1e-08
  Allow_ToCheckOversampling : Inport  Port=2  OutDataTypeStr=boolean  PortDimensions=1  SampleTime=1e-08
  state_edges : Inport  Port=3  OutDataTypeStr=int16  PortDimensions=[4]  SampleTime=1e-08
  omega : Inport  Port=4  OutDataTypeStr=fixdt(1, 24, 11)  PortDimensions=1  SampleTime=1e-08
  OverSamplOmega : Inport  Port=5  OutDataTypeStr=fixdt(1, 24, 11)  PortDimensions=1  SampleTime=1e-08
  Abs : Abs  SampleTime=1e-08  OutDataTypeStr=fixdt(1, 24, 11)  SaturateOnIntegerOverflow=off
  Data Type Conversion1 : DataTypeConversion  OutDataTypeStr=uint16  SampleTime=1e-08  SaturateOnIntegerOverflow=off  RndMeth=Floor
  Delay1 : Delay  DelayLength=double(1)  InitialCondition=0  SampleTime=1e-08
  Delay6 : Delay  DelayLength=double(1)  InitialCondition=0  SampleTime=1e-08
  Delay7 : Delay  DelayLength=double(1)  InitialCondition=1  SampleTime=1e-08
  Sum : Sum  Inputs=+-  AccumDataTypeStr=uint16  OutDataTypeStr=uint16  SampleTime=1e-08
  align_oversamples : Subsystem
  oversample_factor : Subsystem
  oversampling_adjusted : Outport  PortDimensions=4  SampleTime=1e-08
  oversampling_state : Outport  Port=2  SampleTime=1e-08
  wires:
  oversample_factor/2(InternalOmega_Out) -> Delay6/1
  oversample_factor/1(state_Out) -> Delay7/1
  align_oversamples/1(delay_output) -> Delay1/1
  Sum/1 -> oversampling_adjusted/1
  Delay7/1 -> align_oversamples/1(oversampling_factor), oversample_factor/4(state), Data Type Conversion1/1, Sum/1
  Delay6/1 -> oversample_factor/5(InternalOmega)
  Delay1/1 -> Sum/2
  Data Type Conversion1/1 -> oversampling_state/1
  Abs/1 -> oversample_factor/2(ReadBack_Omega)
  OverSamplOmega/1 -> oversample_factor/3(OverSamplOmega)
  omega/1 -> Abs/1
  state_edges/1 -> align_oversamples/3(states)
  Allow_ToCheckOversampling/1 -> oversample_factor/1(AllowCheckOverSampl)
  new_transisiton/1 -> align_oversamples/2(new_transition)
